simulink model "EVdemo_6"  (R2013b)
settings: Solver=FixedStepDiscrete  SolverMode=SingleTasking  StartTime=0.0  StopTime=650  FixedStep=4e-5  MaxStep=1e-5  RelTol=1e-3
InitFcn:
  | %EV_Param_Update
  | % update the number of strings (discretized)
  | numStrings = round(Opti_numStrings);
  | %disp(['Number of strings: ' num2str(numStrings)])
  | % update the effective capacity based on the number of strings
  | EV_Param.Battery_Det.Rated_Capacity = 28.5*numStrings; %A*hr
  | EV_Param.Battery_Det.DP = 1.5*fliplr([1500 1500 1600 1450 1325 1125 925 675 425 175 ])./8*EV_Param.Battery_Det.Rated_Capacity; % 8 comes from the 8Ahr rated batter data used (normalize and rescale to the rated capacity
  | EV_Param.Battery_Det.CP = fliplr([25 100 200 250 375 550 750 950 1125 1150])./8*EV_Param.Battery_Det.Rated_Capacity;
  | 
  | % update the number of cells in a string (discretized)
  | numSeriesCells = round(Opti_numSeriesCells);
  | %disp(['Number of cells in a string: ' num2str(numSeriesCells)])
  | % update the nominal string volage and charge deficit
  | EV_Param.Battery_Det.Nominal_Voltage = numSeriesCells*cellVolts;
  | BatteryParams(1).Qe_init = 0;%EV_Param.Battery_Det.Rated_Capacity*(1-EV_Param.Battery_Det.Initial_SOC/100); %Ampere*hours
  | 
  | % update the total number of cells, battery pack mass and total vehicle
  | % mass
  | total_cells = numSeriesCells*numStrings;
  | %disp(['Total Number of cells: ' num2str(total_cells)])
  | EV_Param.BatteryMass = BatteryParams(1).cell_mass*total_cells;
  | %disp(['Total Battery Pack Mass: ' num2str(EV_Param.BatteryMass)])
  | EV_Param.Vehicle.Mass = 1300+EV_Param.BatteryMass;
  | 
  | % update the driveline gear ratio
  | EV_Param.Vehicle.Engine_Vehicle_Gear_Ratio = Opti_Vehicle_Gear_Ratio;
  | %disp(['Driveline gear ratio: ' num2str(Opti_Vehicle_Gear_Ratio)])
StartFcn:
  | %tic;
StopFcn:
  | %toc;
  | %disp([Final SOC: ' num2str(SOC_final)])
  | %disp([Final Vehicle Error: ' num2str(normed_SQE_final)])
model workspace (MAT data in the model file):
  MCOS : class17 (value not decoded)
  MCOS : class17 (value not decoded)
values from neighbouring files (symbols this model uses):
  Drive_Cycle_Num = 8    [startDemo.m]
undefined symbols (not defined in the file or in its folder): Acc_Cmd, BatteryParams, Brake_Set, cell_area, ctrlConst, current_phase_a, Dec_Cmd, direct_current, DiscIntNeverNeededParam, electromagnetic_torque, HEV_Param, Ion, Kt_Temps, Lithium, Mech_Power_kW, Opti_numSeriesCells, Opti_numStrings, Opti_Vehicle_Gear_Ratio, paramVelocityI, paramVelocityP, paramVelocityPICurrentSat, pmsm, quadrature_current, RLoadLoss, rotor_velocity, sigbuilder_block, Ts, Veh_Spd_Ref
libraries: fl_lib x306, nesl_utility x100, LeadAcidBattery_lib x60, simulink x23, powerlib x16, sdl_lib x7, elec_lib x4, electricdrivelib x2, checkpacklib x2, CustomDriveline_lib x2, LiBatteryBlocks x1, Capacitors_lib x1
(part 6 of 7)

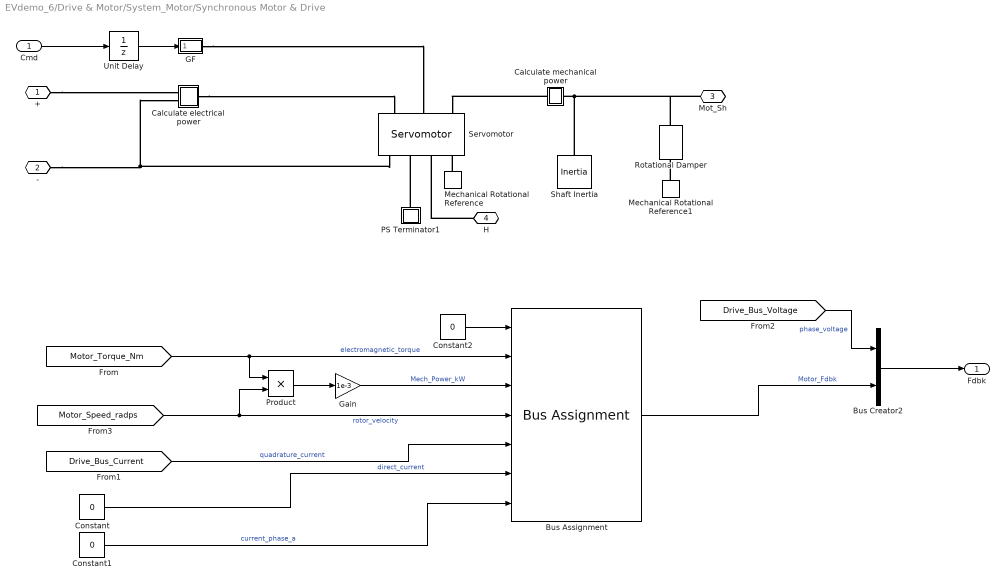
== system EVdemo_6/Drive & Motor/System_Motor/Synchronous Motor & Drive ==
  Cmd : Inport
  Bus Assignment : BusAssignment  AssignedSignals=electromagnetic_torque,Mech_Power_kW,rotor_velocity,quadrature_current,direct_current,current_phase_a
  Bus Creator2 : BusCreator  Inputs=2
  Calculate electrical power : Subsystem
      mask Display: disp('S')
  Calculate mechanical power : Subsystem
      mask Display: disp('S')
  Constant : Constant  Value=0  SampleTime=-1
  Constant1 : Constant  Value=0  SampleTime=-1
  Constant2 : Constant  Value=0  OutDataTypeStr=Bus: Motor_Fdbk  SampleTime=-1
  GF : Subsystem
      mask Display: disp('GF')
  Gain : Gain  Gain=1e-3
  Mechanical Rotational Reference : fl_lib/Mechanical/Rotational Elements/Mechanical Rotational Reference  t_Log=off  LocalVarNames=|t  LocalVarDescs=|t  LocalVarLogging=[]
  Mechanical Rotational Reference1 : fl_lib/Mechanical/Rotational Elements/Mechanical Rotational Reference  t_Log=off  LocalVarNames=|t  LocalVarDescs=|t  LocalVarLogging=0
  PS Terminator1 : Subsystem
      mask Display:
      | plot([0 0.9],[0.5 0.5]);
      | plot([0.5 0.9],[0.3 0.3]);
      | plot([0.5 0.9],[0.7 0.7]);
      | plot([0.9 0.9],[0.7 0.3]);
  Product : Product
  Rotational Damper : fl_lib/Mechanical/Rotational Elements/Rotational Damper  D=EV_Param.Motor.Damping N*m/(rad/s)  t_Log=off  w_Log=off  LocalVarNames=|t|w  LocalVarDescs=|t|w  LocalVarLogging=[0 0]
  Servomotor : elec_lib/Actuators & Drivers/Rotational Actuators/Servomotor  torque_speed_param=1  w_t=EV_Param.Motor.TorqSpdLUT.SpeedRPM rpm  T_t=EV_Param.Motor.TorqSpdLUT.TorqueNm N*m  torque_max=0.1 N*m  power_max=30 W  Tc=EV_Param.Motor.TorqueControl_TimeConst s  eff=EV_Param.Motor.Efficiency  w_eff=4000 rpm  T_eff=280 N*m  Piron=0 W  Pbase=0 W  Res=EV_Param.Motor.Series_Resistance Ohm  J=0 kg*m^2  lam=0 N*m/(rad/s)  speed0=0 rpm  LocalVarLogging=[]  alpha=0.00393 1/K  Tmeas=21 C  thermal_mass=10000 J/K  initial_temperature=21 C
  Shaft Inertia : fl_lib/Mechanical/Rotational Elements/Inertia  inertia=EV_Param.Motor.Shaft_Inertia kg*m^2  initial_velocity=0 rad/s  t_Log=off  LocalVarNames=|t  LocalVarDescs=|t  LocalVarLogging=0
  Unit Delay : UnitDelay  SampleTime=-1
  + : PMIOPort  Port=1  Side=Left
  - : PMIOPort  Port=2  Side=Left
  Mot_Sh : PMIOPort  Port=3  Side=Right
  H : PMIOPort  Port=4  Side=Left
  Fdbk : Outport
  wires:
  Unit Delay/1 -> GF/1(In1)
  Constant1/1 -> Bus Assignment/7  "current_phase_a"
  Constant/1 -> Bus Assignment/6  "direct_current"
  [Drive_Bus_Current] -> Bus Assignment/5  "quadrature_current"
  [Motor_Speed_radps] -> Bus Assignment/4, Product/2  "rotor_velocity"
  [Motor_Torque_Nm] -> Bus Assignment/2, Product/1  "electromagnetic_torque"
  Bus Creator2/1 -> Fdbk/1
  [Drive_Bus_Voltage] -> Bus Creator2/1  "phase_voltage"
  Cmd/1 -> Unit Delay/1
  Product/1 -> Gain/1
  Gain/1 -> Bus Assignment/3  "Mech_Power_kW"
  Constant2/1 -> Bus Assignment/1
  Bus Assignment/1 -> Bus Creator2/2  "Motor_Fdbk"
  connections:
  Mechanical Rotational Reference1/LConn1 -- Rotational Damper/RConn1
  +/RConn1 -- Calculate electrical power/LConn1
  Calculate electrical power/RConn1 -- Servomotor/LConn1
  Shaft Inertia/LConn1 -- Calculate mechanical power/RConn1 -- Rotational Damper/LConn1 -- Mot_Sh/RConn1
  PS Terminator1/LConn1 -- Servomotor/RConn2
  -/RConn1 -- Calculate electrical power/LConn2 -- Servomotor/RConn1
  GF/RConn1 -- Servomotor/LConn2
  Calculate mechanical power/LConn1 -- Servomotor/LConn3
  H/RConn1 -- Servomotor/RConn3
  Mechanical Rotational Reference/LConn1 -- Servomotor/RConn4

== system EVdemo_6/Drive & Motor/System_Motor/ZZZ_Background_Box ==

== system EVdemo_6/Operator Model/Accel_Cmd_Gen/Clamp ==
  preSat : Inport
  saturated : Inport  Port=2
  preIntegrator : Inport  Port=3
  AND : Logic  OutDataTypeStr=boolean
  Compare To Zero : simulink/Logic and Bit Operations/Compare To Zero  relop=<=  OutDataTypeStr=boolean
  Compare To Zero1 : simulink/Logic and Bit Operations/Compare To Zero  relop=<=  OutDataTypeStr=boolean
  Logical Operator : Logic  Operator=NXOR  AllPortsSameDT=off  OutDataTypeStr=boolean
  Clamp : Outport
  wires:
  AND/1 -> Clamp/1
  saturated/1 -> AND/2
  preIntegrator/1 -> Compare To Zero/1
  preSat/1 -> Compare To Zero1/1
  Logical Operator/1 -> AND/1
  Compare To Zero/1 -> Logical Operator/1
  Compare To Zero1/1 -> Logical Operator/2

== system EVdemo_6/Operator Model/Accel_Cmd_Gen/Convert_Data_Type ==
  In1 : Inport
  Data Type Conversion : DataTypeConversion  Priority=27
  Data Type Propagation : simulink/Signal Attributes/Data Type Propagation  Priority=24  PropDataType=fixdt(1, 16)  IfRefDouble=double  IfRefSingle=single  IsSigned=IsSigned1  NumBitsBase=NumBits1  NumBitsMult=1  NumBitsAdd=0  NumBitsAllowFinal=1:128  PropScaling=2^-10  ValuesUsedBestPrec=[5 -7]  SlopeBase=Slope1  SlopeMult=2  SlopeAdd=0  BiasBase=Bias1  BiasMult=1  BiasAdd=0
      settings: AttributesFormatString=-------------------------------\nDT = %<PropDataType>
  Out1 : Outport
  wires:
  In1/1 -> Data Type Propagation/2, Data Type Propagation/1, Data Type Conversion/1
  Data Type Conversion/1 -> Out1/1, Data Type Propagation/3

== system EVdemo_6/Operator Model/Accel_Cmd_Gen/Maintain_Range ==
  In1 : Inport
  Data Type Conversion : DataTypeConversion
  Data Type Propagation : simulink/Signal Attributes/Data Type Propagation  PropDataTypeMode=Specify via dialog  PropDataType=DT_PRECISION_LO  IfRefDouble=double  IfRefSingle=single  IsSigned=IsSigned1  NumBitsBase=NumBits1  NumBitsMult=0  NumBitsAdd=0  NumBitsAllowFinal=1:128  PropScaling=2^-10  ValuesUsedBestPrec=[5 -7]  SlopeBase=PosRange1  SlopeMult=1  SlopeAdd=0  BiasBase=Bias1  BiasMult=1  BiasAdd=0
      settings: AttributesFormatString=-------------------------------\nDT = %<PropDataType>
  Out1 : Outport
  wires:
  In1/1 -> Data Type Propagation/2, Data Type Propagation/1, Data Type Conversion/1
  Data Type Conversion/1 -> Out1/1, Data Type Propagation/3

== system EVdemo_6/Operator Model/Accel_Cmd_Gen/PI_Sat ==
  In1 : Inport
  Constant : Constant  Value=0
  Dynamic Saturation : Subsystem
      mask Display: plot([0.15 0.85],[.5 .5],[.5 .5],[0.05 0.95],0.15+0.7*[0 .25 .75 1],0.05+0.9*[.25 .25 .75 .75]);
  PI_Sat : Constant  Value=EV_Param.Control.Veh_Spd.Sat  PreserveConstantTs=on
  Out1 : Outport
  saturated : Outport  Port=2
  wires:
  Dynamic Saturation/2(sat_mode) -> saturated/1
  Dynamic Saturation/1(y) -> Out1/1
  PI_Sat/1 -> Dynamic Saturation/1(up)
  In1/1 -> Dynamic Saturation/2(u)
  Constant/1 -> Dynamic Saturation/3(lo)

== system EVdemo_6/Operator Model/Brake_Cmd_Gen/Clamp ==
  preSat : Inport
  saturated : Inport  Port=2
  preIntegrator : Inport  Port=3
  AND : Logic  OutDataTypeStr=boolean
  Compare To Zero : simulink/Logic and Bit Operations/Compare To Zero  relop=<=  OutDataTypeStr=boolean
  Compare To Zero1 : simulink/Logic and Bit Operations/Compare To Zero  relop=<=  OutDataTypeStr=boolean
  Logical Operator : Logic  Operator=NXOR  AllPortsSameDT=off  OutDataTypeStr=boolean
  Clamp : Outport
  wires:
  Compare To Zero1/1 -> Logical Operator/2
  Compare To Zero/1 -> Logical Operator/1
  Logical Operator/1 -> AND/1
  preSat/1 -> Compare To Zero1/1
  preIntegrator/1 -> Compare To Zero/1
  saturated/1 -> AND/2
  AND/1 -> Clamp/1

== system EVdemo_6/Operator Model/Brake_Cmd_Gen/Convert_Data_Type ==
  In1 : Inport
  Data Type Conversion : DataTypeConversion  Priority=27
  Data Type Propagation : simulink/Signal Attributes/Data Type Propagation  Priority=24  PropDataType=fixdt(1, 16)  IfRefDouble=double  IfRefSingle=single  IsSigned=IsSigned1  NumBitsBase=NumBits1  NumBitsMult=1  NumBitsAdd=0  NumBitsAllowFinal=1:128  PropScaling=2^-10  ValuesUsedBestPrec=[5 -7]  SlopeBase=Slope1  SlopeMult=2  SlopeAdd=0  BiasBase=Bias1  BiasMult=1  BiasAdd=0
      settings: AttributesFormatString=-------------------------------\nDT = %<PropDataType>
  Out1 : Outport
  wires:
  Data Type Conversion/1 -> Data Type Propagation/3, Out1/1
  In1/1 -> Data Type Conversion/1, Data Type Propagation/1, Data Type Propagation/2

== system EVdemo_6/Operator Model/Brake_Cmd_Gen/Maintain_Range ==
  In1 : Inport
  Data Type Conversion : DataTypeConversion
  Data Type Propagation : simulink/Signal Attributes/Data Type Propagation  PropDataTypeMode=Specify via dialog  PropDataType=DT_PRECISION_LO  IfRefDouble=double  IfRefSingle=single  IsSigned=IsSigned1  NumBitsBase=NumBits1  NumBitsMult=0  NumBitsAdd=0  NumBitsAllowFinal=1:128  PropScaling=2^-10  ValuesUsedBestPrec=[5 -7]  SlopeBase=PosRange1  SlopeMult=1  SlopeAdd=0  BiasBase=Bias1  BiasMult=1  BiasAdd=0
      settings: AttributesFormatString=-------------------------------\nDT = %<PropDataType>
  Out1 : Outport
  wires:
  Data Type Conversion/1 -> Data Type Propagation/3, Out1/1
  In1/1 -> Data Type Conversion/1, Data Type Propagation/1, Data Type Propagation/2

== system EVdemo_6/Operator Model/Brake_Cmd_Gen/PI_Sat ==
  In1 : Inport
  Constant : Constant  Value=0
  Dynamic Saturation : Subsystem
      mask Display: plot([0.15 0.85],[.5 .5],[.5 .5],[0.05 0.95],0.15+0.7*[0 .25 .75 1],0.05+0.9*[.25 .25 .75 .75]);
  PI_Sat : Constant  Value=-EV_Param.Control.Veh_Brake.Sat  PreserveConstantTs=on
  Out1 : Outport
  saturated : Outport  Port=2
  wires:
  Constant/1 -> Dynamic Saturation/1(up)
  In1/1 -> Dynamic Saturation/2(u)
  PI_Sat/1 -> Dynamic Saturation/3(lo)
  Dynamic Saturation/1(y) -> Out1/1
  Dynamic Saturation/2(sat_mode) -> saturated/1

== system EVdemo_6/Vehicle/Full/2nd Order LP Filter (Butterworth) ==
  u : Inport
  Spd_Err_Filt_BW [rad/s] : Inport  Port=2
  -1 : Gain  Gain=-1
  -1.4142/(Spd_Err_Filt_BW) : Gain  Gain=-1.4142
  Add4 : Sum  Inputs=+++
  Compare To Zero : simulink/Logic and Bit Operations/Compare To Zero  relop=<=  OutDataTypeStr=uint8
  Discrete-Time Integrator : DiscreteIntegrator  ExternalReset=rising  SampleTime=DT  ICPrevOutput=DiscIntNeverNeededParam  ICPrevScaledInput=DiscIntNeverNeededParam
  Discrete-Time Integrator1 : DiscreteIntegrator  ExternalReset=rising  SampleTime=DT  ICPrevOutput=DiscIntNeverNeededParam  ICPrevScaledInput=DiscIntNeverNeededParam
  Math Function : Math  Operator=square  SaturateOnIntegerOverflow=on
  Product : Product  RndMeth=Zero
  Product1 : Product  Inputs=*/  RndMeth=Zero
  Saturation1 : Saturate  UpperLimit=2*pi*5000  LowerLimit=.001
  y : Outport
  wires:
  Add4/1 -> Product/2
  Discrete-Time Integrator/1 -> Product1/1, Discrete-Time Integrator1/1  "X_1"
  Discrete-Time Integrator1/1 -> -1/1, y/1  "x_2"
  -1.4142/(Spd_Err_Filt_BW)/1 -> Add4/3
  -1/1 -> Add4/2
  Product/1 -> Discrete-Time Integrator/1  "x_0"
  u/1 -> Add4/1
  Math Function/1 -> Product/1, Compare To Zero/1
  Spd_Err_Filt_BW [rad/s]/1 -> Saturation1/1
  Product1/1 -> -1.4142/(Spd_Err_Filt_BW)/1
  Compare To Zero/1 -> Discrete-Time Integrator/2, Discrete-Time Integrator1/2
  Saturation1/1 -> Math Function/1, Product1/2

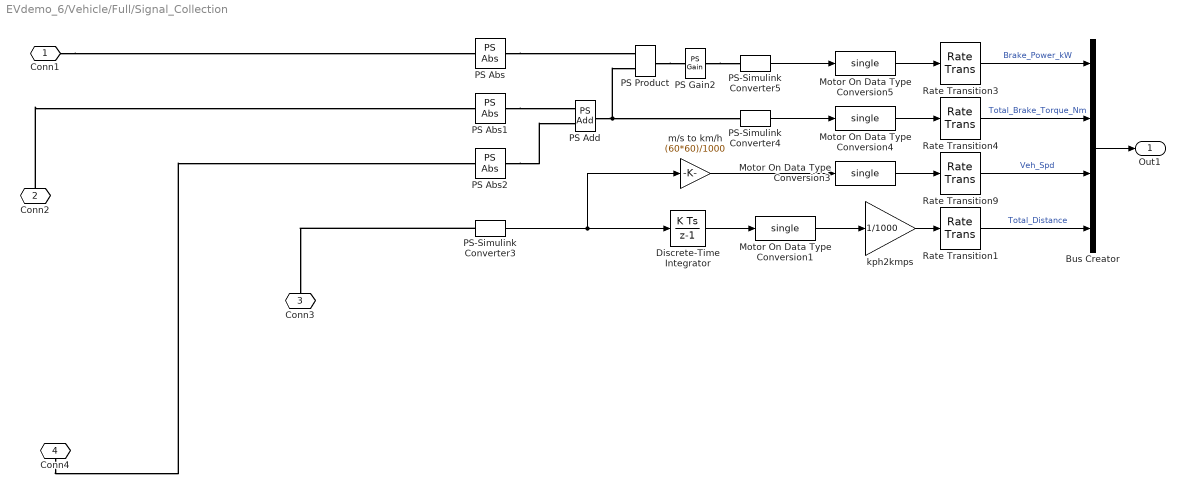
== system EVdemo_6/Vehicle/Full/Signal_Collection ==
  Bus Creator : BusCreator
  Discrete-Time Integrator : DiscreteIntegrator  SampleTime=-1  ICPrevOutput=DiscIntNeverNeededParam  ICPrevScaledInput=DiscIntNeverNeededParam
  Motor On Data Type Conversion{1,3..5} (4 alike) : DataTypeConversion  OutDataTypeStr=single
  PS Abs : fl_lib/Physical Signals/Nonlinear Operators/PS Abs  LocalVarLogging=[]
  PS Abs1 : fl_lib/Physical Signals/Nonlinear Operators/PS Abs  LocalVarLogging=[]
  PS Abs2 : fl_lib/Physical Signals/Nonlinear Operators/PS Abs  LocalVarLogging=[]
  PS Add : fl_lib/Physical Signals/Functions/PS Add  LocalVarLogging=[]
  PS Gain2 : fl_lib/Physical Signals/Functions/PS Gain  gain=1e-3  LocalVarLogging=[]
  PS Product : fl_lib/Physical Signals/Functions/PS Product  LocalVarLogging=[]
  PS-Simulink Converter3 : nesl_utility/PS-Simulink Converter  PhysicalDomain=network_engine_domain  SubClassName=ps_output  LeftPortType=input  RightPortType=output  PseudoPeriodic=off  Frequencies=[]  Unit=m/s  AffineConversion=off
  PS-Simulink Converter4 : nesl_utility/PS-Simulink Converter  PhysicalDomain=network_engine_domain  SubClassName=ps_output  LeftPortType=input  RightPortType=output  PseudoPeriodic=off  Frequencies=[]  Unit=m/s  AffineConversion=off
  PS-Simulink Converter5 : nesl_utility/PS-Simulink Converter  PhysicalDomain=network_engine_domain  SubClassName=ps_output  LeftPortType=input  RightPortType=output  PseudoPeriodic=off  Frequencies=[]  Unit=m/s  AffineConversion=off
  Rate Transition{1,3..4,9} (4 alike) : RateTransition  OutPortSampleTime=.01
  kph2kmps : Gain  Gain=1/1000
  m/s to km/h : Gain  Gain=(60*60)/1000
  Conn1 : PMIOPort  Port=1  Side=Left
  Conn2 : PMIOPort  Port=2  Side=Left
  Conn3 : PMIOPort  Port=3  Side=Left
  Conn4 : PMIOPort  Port=4  Side=Left
  Out1 : Outport
  wires:
  PS-Simulink Converter4/1 -> Motor On Data Type Conversion4/1
  PS-Simulink Converter5/1 -> Motor On Data Type Conversion5/1
  Rate Transition3/1 -> Bus Creator/1  "Brake_Power_kW"
  Rate Transition4/1 -> Bus Creator/2  "Total_Brake_Torque_Nm"
  Motor On Data Type Conversion4/1 -> Rate Transition4/1
  Motor On Data Type Conversion5/1 -> Rate Transition3/1
  Discrete-Time Integrator/1 -> Motor On Data Type Conversion1/1
  m/s to km/h/1 -> Motor On Data Type Conversion3/1
  Motor On Data Type Conversion3/1 -> Rate Transition9/1
  kph2kmps/1 -> Rate Transition1/1
  Rate Transition1/1 -> Bus Creator/4  "Total_Distance"
  Bus Creator/1 -> Out1/1
  Motor On Data Type Conversion1/1 -> kph2kmps/1
  Rate Transition9/1 -> Bus Creator/3  "Veh_Spd"
  PS-Simulink Converter3/1 -> m/s to km/h/1, Discrete-Time Integrator/1
  connections:
  PS Abs/RConn1 -- PS Product/LConn1
  PS Product/RConn1 -- PS Gain2/LConn1
  PS Gain2/RConn1 -- PS-Simulink Converter5/LConn1
  PS Abs1/RConn1 -- PS Add/LConn1
  PS Abs2/RConn1 -- PS Add/LConn2
  Conn1/RConn1 -- PS Abs/LConn1
  PS Add/RConn1 -- PS Product/LConn2 -- PS-Simulink Converter4/LConn1
  Conn2/RConn1 -- PS Abs1/LConn1
  Conn4/RConn1 -- PS Abs2/LConn1
  PS-Simulink Converter3/LConn1 -- Conn3/RConn1

== system EVdemo_6/Vehicle/Full/Vehicle Speed, Power ==
  Ideal Rotational Motion Sensor : fl_lib/Mechanical/Mechanical Sensors/Ideal Rotational Motion Sensor  offset=0 rad  w_Log=off  t_Log=off  phi_Log=off  LocalVarNames=|w|t|phi  LocalVarDescs=|w|t|phi  LocalVarLogging=[0 0 0]
  Ideal Torque Sensor : fl_lib/Mechanical/Mechanical Sensors/Ideal Torque Sensor  w_Log=off  t_Log=off  LocalVarNames=|w|t  LocalVarDescs=|w|t  LocalVarLogging=[0 0]
  Mechanical Rotational Reference : fl_lib/Mechanical/Rotational Elements/Mechanical Rotational Reference  t_Log=off  LocalVarNames=|t  LocalVarDescs=|t  LocalVarLogging=0
  PS-Simulink Converter : nesl_utility/PS-Simulink Converter  PhysicalDomain=network_engine_domain  SubClassName=ps_output  LeftPortType=input  RightPortType=output  PseudoPeriodic=off  Frequencies=[]  Unit=N*m  AffineConversion=off
  PS-Simulink Converter1 : nesl_utility/PS-Simulink Converter  PhysicalDomain=network_engine_domain  SubClassName=ps_output  LeftPortType=input  RightPortType=output  PseudoPeriodic=off  Frequencies=[]  Unit=rad/s  AffineConversion=off
  Product : Product  RndMeth=Zero
  W2kW : Gain  Gain=0.001
  B : PMIOPort  Port=1  Side=Left
  F : PMIOPort  Port=2  Side=Right
  tag scope: Pm_vehicle=global
  wires:
  PS-Simulink Converter1/1 -> Product/2
  PS-Simulink Converter/1 -> Product/1
  Product/1 -> W2kW/1
  W2kW/1 -> [Pm_vehicle]
  connections:
  PS-Simulink Converter1/LConn1 -- Ideal Rotational Motion Sensor/RConn2
  PS-Simulink Converter/LConn1 -- Ideal Torque Sensor/RConn2
  B/RConn1 -- Ideal Torque Sensor/LConn1
  Ideal Torque Sensor/RConn1 -- F/RConn1 -- Ideal Rotational Motion Sensor/LConn1
  Mechanical Rotational Reference/LConn1 -- Ideal Rotational Motion Sensor/RConn1

== system EVdemo_6/Vehicle/Simple/Aerodynamic Drag ==
  Cd1 : fl_lib/Physical Signals/Functions/PS Gain  gain=Cd  LocalVarLogging=[]
  PS Math Function : fl_lib/Physical Signals/Functions/PS Math Function  fcn_choice=7  LocalVarLogging=[]
  PS Product : fl_lib/Physical Signals/Functions/PS Product  LocalVarLogging=[]
  PS Sign : fl_lib/Physical Signals/Nonlinear Operators/PS Sign  LocalVarLogging=[]
  half1 : fl_lib/Physical Signals/Functions/PS Gain  gain=1/2  LocalVarLogging=[]
  kph to mps1 : fl_lib/Physical Signals/Functions/PS Gain  gain=1/3.6  LocalVarLogging=[]
  radius1 : fl_lib/Physical Signals/Functions/PS Gain  gain=-radius  LocalVarLogging=[]
  Conn1 : PMIOPort  Port=1  Side=Left
  Conn2 : PMIOPort  Port=2  Side=Right
  connections:
  PS Sign/RConn1 -- PS Product/LConn2
  radius1/LConn1 -- Cd1/RConn1
  radius1/RConn1 -- PS Product/LConn1
  Cd1/LConn1 -- half1/RConn1
  PS Math Function/LConn1 -- kph to mps1/RConn1
  half1/LConn1 -- PS Math Function/RConn1
  kph to mps1/LConn1 -- PS Sign/LConn1 -- Conn1/RConn1
  Conn2/RConn1 -- PS Product/RConn1

== system EVdemo_6/Vehicle/Simple/Vehicle Speed, Power ==
  Ideal Rotational Motion Sensor : fl_lib/Mechanical/Mechanical Sensors/Ideal Rotational Motion Sensor  offset=0 rad  w_Log=off  t_Log=off  phi_Log=off  LocalVarNames=|w|t|phi  LocalVarDescs=|w|t|phi  LocalVarLogging=[0 0 0]
  Ideal Torque Sensor : fl_lib/Mechanical/Mechanical Sensors/Ideal Torque Sensor  w_Log=off  t_Log=off  LocalVarNames=|w|t  LocalVarDescs=|w|t  LocalVarLogging=[0 0]
  Mechanical Rotational Reference : fl_lib/Mechanical/Rotational Elements/Mechanical Rotational Reference  t_Log=off  LocalVarNames=|t  LocalVarDescs=|t  LocalVarLogging=0
  PS-Simulink Converter : nesl_utility/PS-Simulink Converter  PhysicalDomain=network_engine_domain  SubClassName=ps_output  LeftPortType=input  RightPortType=output  PseudoPeriodic=off  Frequencies=[]  Unit=N*m  AffineConversion=off
  PS-Simulink Converter1 : nesl_utility/PS-Simulink Converter  PhysicalDomain=network_engine_domain  SubClassName=ps_output  LeftPortType=input  RightPortType=output  PseudoPeriodic=off  Frequencies=[]  Unit=rad/s  AffineConversion=off
  Product : Product  RndMeth=Zero
  W2kW : Gain  Gain=0.001
  rad/s to km/h : fl_lib/Physical Signals/Functions/PS Gain  gain=radius*3.6  LocalVarLogging=[]
  B : PMIOPort  Port=1  Side=Left
  F : PMIOPort  Port=2  Side=Left
  Speed : PMIOPort  Port=3  Side=Right
  tag scope: Pm_vehicle=global
  wires:
  W2kW/1 -> [Pm_vehicle]
  Product/1 -> W2kW/1
  PS-Simulink Converter/1 -> Product/1
  PS-Simulink Converter1/1 -> Product/2
  connections:
  Mechanical Rotational Reference/LConn1 -- Ideal Rotational Motion Sensor/RConn1
  Ideal Rotational Motion Sensor/LConn1 -- F/RConn1 -- Ideal Torque Sensor/RConn1
  B/RConn1 -- Ideal Torque Sensor/LConn1
  PS-Simulink Converter/LConn1 -- Ideal Torque Sensor/RConn2
  rad/s to km/h/LConn1 -- Ideal Rotational Motion Sensor/RConn2 -- PS-Simulink Converter1/LConn1
  Speed/RConn1 -- rad/s to km/h/RConn1

== system EVdemo_6/Battery/Cells/Battery cell1/ DOC  ==
  PS-Simulink Converter1 : nesl_utility/PS-Simulink Converter  PhysicalDomain=network_engine_domain  SubClassName=ps_output  LeftPortType=input  RightPortType=output  PseudoPeriodic=off  Frequencies=[]  Unit=1  AffineConversion=off
  PS : PMIOPort  Port=1  Side=Left
  tag scope: DOC=global
  wires:
  PS-Simulink Converter1/1 -> [DOC]
  connections:
  PS/RConn1 -- PS-Simulink Converter1/LConn1

== system EVdemo_6/Battery/Cells/Battery cell1/ SOC  ==
  PS-Simulink Converter1 : nesl_utility/PS-Simulink Converter  PhysicalDomain=network_engine_domain  SubClassName=ps_output  LeftPortType=input  RightPortType=output  PseudoPeriodic=off  Frequencies=[]  Unit=1  AffineConversion=off
  PS : PMIOPort  Port=1  Side=Left
  tag scope: SOC=global
  wires:
  PS-Simulink Converter1/1 -> [SOC]
  connections:
  PS/RConn1 -- PS-Simulink Converter1/LConn1

== system EVdemo_6/Battery/Cells/Battery cell1/T ==
  PS-Simulink Converter1 : nesl_utility/PS-Simulink Converter  PhysicalDomain=network_engine_domain  SubClassName=ps_output  LeftPortType=input  RightPortType=output  PseudoPeriodic=off  Frequencies=[]  Unit=C  AffineConversion=on
  PS : PMIOPort  Port=1  Side=Left
  tag scope: Batt_Cell_Temp=global
  wires:
  PS-Simulink Converter1/1 -> [Batt_Cell_Temp]
  connections:
  PS/RConn1 -- PS-Simulink Converter1/LConn1

== system EVdemo_6/Battery/Cells/Battery cell1/Thermal Model ==
  Battery thermal mass : fl_lib/Thermal/Thermal Elements/Thermal Mass  mass=1 kg  sp_heat=HEV_Param.Battery_Cell.Ctheta J/kg/K  init_temp=HEV_Param.Battery_Cell.theta_init+273 K  Q_Log=off  LocalVarNames=|heat_flow|temperature  LocalVarDescs=|Heat flow (J/s)|Mass temperature (K)  LocalVarLogging=[0 0]
  Ideal Temperature Sensor : fl_lib/Thermal/Thermal Sensors/Ideal Temperature Sensor  Qs_Log=off  Ts_Log=off  LocalVarNames=|Qs|Ts  LocalVarDescs=|Qs|Ts  LocalVarLogging=[]
  Ideal Heat Flow Source : fl_lib/Thermal/Thermal Sources/Ideal Heat Flow Source  Q_Log=off  T_Log=off  LocalVarNames=|heat_flow|T_differential  LocalVarDescs=|Heat flow through the source (J/s)|Temperature differential across the source (K)  LocalVarLogging=[0 0]
  Kt as a function of temperature : fl_lib/Physical Signals/Lookup Tables/PS Lookup Table (1D)  x_t=[HEV_Param.Battery_Cell.theta_f,HEV_Param.Battery_Cell. Kt_Temps]+273  y_t=[0 HEV_Param.Battery_Cell.Kt]  interp_method=1  extrap_method=1  LocalVarLogging=[]
  Thermal Reference1 : fl_lib/Thermal/Thermal Elements/Thermal Reference  Q_Log=off  LocalVarNames=|Q  LocalVarDescs=|Q  LocalVarLogging=[]
  Thermal Reference2 : fl_lib/Thermal/Thermal Elements/Thermal Reference  Q_Log=off  LocalVarNames=|Q  LocalVarDescs=|Q  LocalVarLogging=[]
  Ps : PMIOPort  Tag=PMCPort  Port=1  Side=Left
  H : PMIOPort  Tag=PMCPort  Port=2  Side=Left
  Kt : PMIOPort  Tag=PMCPort  Port=3  Side=Right
  T : PMIOPort  Tag=PMCPort  Port=4  Side=Right
  connections:
  Ideal Heat Flow Source/RConn1 -- Ps/RConn1
  Kt/RConn1 -- Kt as a function of temperature/RConn1
  Battery thermal mass/LConn1 -- Ideal Heat Flow Source/LConn1 -- Ideal Temperature Sensor/LConn1 -- H/RConn1
  Thermal Reference1/LConn1 -- Ideal Heat Flow Source/RConn2
  T/RConn1 -- Kt as a function of temperature/LConn1 -- Ideal Temperature Sensor/RConn2
  Ideal Temperature Sensor/RConn1 -- Thermal Reference2/LConn1

== system EVdemo_6/Battery/Cells/Battery cell10/Thermal Model ==
  Battery thermal mass : fl_lib/Thermal/Thermal Elements/Thermal Mass  mass=1 kg  sp_heat=HEV_Param.Battery_Cell.Ctheta J/kg/K  init_temp=HEV_Param.Battery_Cell.theta_init+273 K  Q_Log=off  LocalVarNames=|heat_flow|temperature  LocalVarDescs=|Heat flow (J/s)|Mass temperature (K)  LocalVarLogging=[0 0]
  Ideal Temperature Sensor : fl_lib/Thermal/Thermal Sensors/Ideal Temperature Sensor  Qs_Log=off  Ts_Log=off  LocalVarNames=|Qs|Ts  LocalVarDescs=|Qs|Ts  LocalVarLogging=[]
  Ideal Heat Flow Source : fl_lib/Thermal/Thermal Sources/Ideal Heat Flow Source  Q_Log=off  T_Log=off  LocalVarNames=|heat_flow|T_differential  LocalVarDescs=|Heat flow through the source (J/s)|Temperature differential across the source (K)  LocalVarLogging=[0 0]
  Kt as a function of temperature : fl_lib/Physical Signals/Lookup Tables/PS Lookup Table (1D)  x_t=[HEV_Param.Battery_Cell.theta_f,HEV_Param.Battery_Cell. Kt_Temps]+273  y_t=[0 HEV_Param.Battery_Cell.Kt]  interp_method=1  extrap_method=1  LocalVarLogging=[]
  Thermal Reference1 : fl_lib/Thermal/Thermal Elements/Thermal Reference  Q_Log=off  LocalVarNames=|Q  LocalVarDescs=|Q  LocalVarLogging=[]
  Thermal Reference2 : fl_lib/Thermal/Thermal Elements/Thermal Reference  Q_Log=off  LocalVarNames=|Q  LocalVarDescs=|Q  LocalVarLogging=[]
  Ps : PMIOPort  Tag=PMCPort  Port=1  Side=Left
  H : PMIOPort  Tag=PMCPort  Port=2  Side=Left
  Kt : PMIOPort  Tag=PMCPort  Port=3  Side=Right
  T : PMIOPort  Tag=PMCPort  Port=4  Side=Right
  connections:
  Ideal Heat Flow Source/RConn1 -- Ps/RConn1
  Kt/RConn1 -- Kt as a function of temperature/RConn1
  Battery thermal mass/LConn1 -- Ideal Heat Flow Source/LConn1 -- Ideal Temperature Sensor/LConn1 -- H/RConn1
  Thermal Reference1/LConn1 -- Ideal Heat Flow Source/RConn2
  T/RConn1 -- Kt as a function of temperature/LConn1 -- Ideal Temperature Sensor/RConn2
  Ideal Temperature Sensor/RConn1 -- Thermal Reference2/LConn1

== system EVdemo_6/Battery/Cells/Battery cell2/Thermal Model ==
  Battery thermal mass : fl_lib/Thermal/Thermal Elements/Thermal Mass  mass=1 kg  sp_heat=HEV_Param.Battery_Cell.Ctheta J/kg/K  init_temp=HEV_Param.Battery_Cell.theta_init+273 K  Q_Log=off  LocalVarNames=|heat_flow|temperature  LocalVarDescs=|Heat flow (J/s)|Mass temperature (K)  LocalVarLogging=[0 0]
  Ideal Temperature Sensor : fl_lib/Thermal/Thermal Sensors/Ideal Temperature Sensor  Qs_Log=off  Ts_Log=off  LocalVarNames=|Qs|Ts  LocalVarDescs=|Qs|Ts  LocalVarLogging=[]
  Ideal Heat Flow Source : fl_lib/Thermal/Thermal Sources/Ideal Heat Flow Source  Q_Log=off  T_Log=off  LocalVarNames=|heat_flow|T_differential  LocalVarDescs=|Heat flow through the source (J/s)|Temperature differential across the source (K)  LocalVarLogging=[0 0]
  Kt as a function of temperature : fl_lib/Physical Signals/Lookup Tables/PS Lookup Table (1D)  x_t=[HEV_Param.Battery_Cell.theta_f,HEV_Param.Battery_Cell. Kt_Temps]+273  y_t=[0 HEV_Param.Battery_Cell.Kt]  interp_method=1  extrap_method=1  LocalVarLogging=[]
  Thermal Reference1 : fl_lib/Thermal/Thermal Elements/Thermal Reference  Q_Log=off  LocalVarNames=|Q  LocalVarDescs=|Q  LocalVarLogging=[]
  Thermal Reference2 : fl_lib/Thermal/Thermal Elements/Thermal Reference  Q_Log=off  LocalVarNames=|Q  LocalVarDescs=|Q  LocalVarLogging=[]
  Ps : PMIOPort  Tag=PMCPort  Port=1  Side=Left
  H : PMIOPort  Tag=PMCPort  Port=2  Side=Left
  Kt : PMIOPort  Tag=PMCPort  Port=3  Side=Right
  T : PMIOPort  Tag=PMCPort  Port=4  Side=Right
  connections:
  Ideal Temperature Sensor/RConn1 -- Thermal Reference2/LConn1
  Ideal Temperature Sensor/RConn2 -- Kt as a function of temperature/LConn1 -- T/RConn1
  Thermal Reference1/LConn1 -- Ideal Heat Flow Source/RConn2
  H/RConn1 -- Ideal Temperature Sensor/LConn1 -- Ideal Heat Flow Source/LConn1 -- Battery thermal mass/LConn1
  Kt/RConn1 -- Kt as a function of temperature/RConn1
  Ideal Heat Flow Source/RConn1 -- Ps/RConn1

== system EVdemo_6/Battery/Cells/Battery cell3/Thermal Model ==
  Battery thermal mass : fl_lib/Thermal/Thermal Elements/Thermal Mass  mass=1 kg  sp_heat=HEV_Param.Battery_Cell.Ctheta J/kg/K  init_temp=HEV_Param.Battery_Cell.theta_init+273 K  Q_Log=off  LocalVarNames=|heat_flow|temperature  LocalVarDescs=|Heat flow (J/s)|Mass temperature (K)  LocalVarLogging=[0 0]
  Ideal Temperature Sensor : fl_lib/Thermal/Thermal Sensors/Ideal Temperature Sensor  Qs_Log=off  Ts_Log=off  LocalVarNames=|Qs|Ts  LocalVarDescs=|Qs|Ts  LocalVarLogging=[]
  Ideal Heat Flow Source : fl_lib/Thermal/Thermal Sources/Ideal Heat Flow Source  Q_Log=off  T_Log=off  LocalVarNames=|heat_flow|T_differential  LocalVarDescs=|Heat flow through the source (J/s)|Temperature differential across the source (K)  LocalVarLogging=[0 0]
  Kt as a function of temperature : fl_lib/Physical Signals/Lookup Tables/PS Lookup Table (1D)  x_t=[HEV_Param.Battery_Cell.theta_f,HEV_Param.Battery_Cell. Kt_Temps]+273  y_t=[0 HEV_Param.Battery_Cell.Kt]  interp_method=1  extrap_method=1  LocalVarLogging=[]
  Thermal Reference1 : fl_lib/Thermal/Thermal Elements/Thermal Reference  Q_Log=off  LocalVarNames=|Q  LocalVarDescs=|Q  LocalVarLogging=[]
  Thermal Reference2 : fl_lib/Thermal/Thermal Elements/Thermal Reference  Q_Log=off  LocalVarNames=|Q  LocalVarDescs=|Q  LocalVarLogging=[]
  Ps : PMIOPort  Tag=PMCPort  Port=1  Side=Left
  H : PMIOPort  Tag=PMCPort  Port=2  Side=Left
  Kt : PMIOPort  Tag=PMCPort  Port=3  Side=Right
  T : PMIOPort  Tag=PMCPort  Port=4  Side=Right
  connections:
  Ideal Heat Flow Source/RConn1 -- Ps/RConn1
  Kt/RConn1 -- Kt as a function of temperature/RConn1
  Battery thermal mass/LConn1 -- Ideal Heat Flow Source/LConn1 -- Ideal Temperature Sensor/LConn1 -- H/RConn1
  Thermal Reference1/LConn1 -- Ideal Heat Flow Source/RConn2
  T/RConn1 -- Kt as a function of temperature/LConn1 -- Ideal Temperature Sensor/RConn2
  Ideal Temperature Sensor/RConn1 -- Thermal Reference2/LConn1

== system EVdemo_6/Battery/Cells/Battery cell4/Thermal Model ==
  Battery thermal mass : fl_lib/Thermal/Thermal Elements/Thermal Mass  mass=1 kg  sp_heat=HEV_Param.Battery_Cell.Ctheta J/kg/K  init_temp=HEV_Param.Battery_Cell.theta_init+273 K  Q_Log=off  LocalVarNames=|heat_flow|temperature  LocalVarDescs=|Heat flow (J/s)|Mass temperature (K)  LocalVarLogging=[0 0]
  Ideal Temperature Sensor : fl_lib/Thermal/Thermal Sensors/Ideal Temperature Sensor  Qs_Log=off  Ts_Log=off  LocalVarNames=|Qs|Ts  LocalVarDescs=|Qs|Ts  LocalVarLogging=[]
  Ideal Heat Flow Source : fl_lib/Thermal/Thermal Sources/Ideal Heat Flow Source  Q_Log=off  T_Log=off  LocalVarNames=|heat_flow|T_differential  LocalVarDescs=|Heat flow through the source (J/s)|Temperature differential across the source (K)  LocalVarLogging=[0 0]
  Kt as a function of temperature : fl_lib/Physical Signals/Lookup Tables/PS Lookup Table (1D)  x_t=[HEV_Param.Battery_Cell.theta_f,HEV_Param.Battery_Cell. Kt_Temps]+273  y_t=[0 HEV_Param.Battery_Cell.Kt]  interp_method=1  extrap_method=1  LocalVarLogging=[]
  Thermal Reference1 : fl_lib/Thermal/Thermal Elements/Thermal Reference  Q_Log=off  LocalVarNames=|Q  LocalVarDescs=|Q  LocalVarLogging=[]
  Thermal Reference2 : fl_lib/Thermal/Thermal Elements/Thermal Reference  Q_Log=off  LocalVarNames=|Q  LocalVarDescs=|Q  LocalVarLogging=[]
  Ps : PMIOPort  Tag=PMCPort  Port=1  Side=Left
  H : PMIOPort  Tag=PMCPort  Port=2  Side=Left
  Kt : PMIOPort  Tag=PMCPort  Port=3  Side=Right
  T : PMIOPort  Tag=PMCPort  Port=4  Side=Right
  connections:
  Ideal Heat Flow Source/RConn1 -- Ps/RConn1
  Kt/RConn1 -- Kt as a function of temperature/RConn1
  Battery thermal mass/LConn1 -- Ideal Heat Flow Source/LConn1 -- Ideal Temperature Sensor/LConn1 -- H/RConn1
  Thermal Reference1/LConn1 -- Ideal Heat Flow Source/RConn2
  T/RConn1 -- Kt as a function of temperature/LConn1 -- Ideal Temperature Sensor/RConn2
  Ideal Temperature Sensor/RConn1 -- Thermal Reference2/LConn1

== system EVdemo_6/Battery/Cells/Battery cell5/Thermal Model ==
  Battery thermal mass : fl_lib/Thermal/Thermal Elements/Thermal Mass  mass=1 kg  sp_heat=HEV_Param.Battery_Cell.Ctheta J/kg/K  init_temp=HEV_Param.Battery_Cell.theta_init+273 K  Q_Log=off  LocalVarNames=|heat_flow|temperature  LocalVarDescs=|Heat flow (J/s)|Mass temperature (K)  LocalVarLogging=[0 0]
  Ideal Temperature Sensor : fl_lib/Thermal/Thermal Sensors/Ideal Temperature Sensor  Qs_Log=off  Ts_Log=off  LocalVarNames=|Qs|Ts  LocalVarDescs=|Qs|Ts  LocalVarLogging=[]
  Ideal Heat Flow Source : fl_lib/Thermal/Thermal Sources/Ideal Heat Flow Source  Q_Log=off  T_Log=off  LocalVarNames=|heat_flow|T_differential  LocalVarDescs=|Heat flow through the source (J/s)|Temperature differential across the source (K)  LocalVarLogging=[0 0]
  Kt as a function of temperature : fl_lib/Physical Signals/Lookup Tables/PS Lookup Table (1D)  x_t=[HEV_Param.Battery_Cell.theta_f,HEV_Param.Battery_Cell. Kt_Temps]+273  y_t=[0 HEV_Param.Battery_Cell.Kt]  interp_method=1  extrap_method=1  LocalVarLogging=[]
  Thermal Reference1 : fl_lib/Thermal/Thermal Elements/Thermal Reference  Q_Log=off  LocalVarNames=|Q  LocalVarDescs=|Q  LocalVarLogging=[]
  Thermal Reference2 : fl_lib/Thermal/Thermal Elements/Thermal Reference  Q_Log=off  LocalVarNames=|Q  LocalVarDescs=|Q  LocalVarLogging=[]
  Ps : PMIOPort  Tag=PMCPort  Port=1  Side=Left
  H : PMIOPort  Tag=PMCPort  Port=2  Side=Left
  Kt : PMIOPort  Tag=PMCPort  Port=3  Side=Right
  T : PMIOPort  Tag=PMCPort  Port=4  Side=Right
  connections:
  Ideal Heat Flow Source/RConn1 -- Ps/RConn1
  Kt/RConn1 -- Kt as a function of temperature/RConn1
  Battery thermal mass/LConn1 -- Ideal Heat Flow Source/LConn1 -- Ideal Temperature Sensor/LConn1 -- H/RConn1
  Thermal Reference1/LConn1 -- Ideal Heat Flow Source/RConn2
  T/RConn1 -- Kt as a function of temperature/LConn1 -- Ideal Temperature Sensor/RConn2
  Ideal Temperature Sensor/RConn1 -- Thermal Reference2/LConn1

== system EVdemo_6/Battery/Cells/Battery cell6/Thermal Model ==
  Battery thermal mass : fl_lib/Thermal/Thermal Elements/Thermal Mass  mass=1 kg  sp_heat=HEV_Param.Battery_Cell.Ctheta J/kg/K  init_temp=HEV_Param.Battery_Cell.theta_init+273 K  Q_Log=off  LocalVarNames=|heat_flow|temperature  LocalVarDescs=|Heat flow (J/s)|Mass temperature (K)  LocalVarLogging=[0 0]
  Ideal Temperature Sensor : fl_lib/Thermal/Thermal Sensors/Ideal Temperature Sensor  Qs_Log=off  Ts_Log=off  LocalVarNames=|Qs|Ts  LocalVarDescs=|Qs|Ts  LocalVarLogging=[]
  Ideal Heat Flow Source : fl_lib/Thermal/Thermal Sources/Ideal Heat Flow Source  Q_Log=off  T_Log=off  LocalVarNames=|heat_flow|T_differential  LocalVarDescs=|Heat flow through the source (J/s)|Temperature differential across the source (K)  LocalVarLogging=[0 0]
  Kt as a function of temperature : fl_lib/Physical Signals/Lookup Tables/PS Lookup Table (1D)  x_t=[HEV_Param.Battery_Cell.theta_f,HEV_Param.Battery_Cell. Kt_Temps]+273  y_t=[0 HEV_Param.Battery_Cell.Kt]  interp_method=1  extrap_method=1  LocalVarLogging=[]
  Thermal Reference1 : fl_lib/Thermal/Thermal Elements/Thermal Reference  Q_Log=off  LocalVarNames=|Q  LocalVarDescs=|Q  LocalVarLogging=[]
  Thermal Reference2 : fl_lib/Thermal/Thermal Elements/Thermal Reference  Q_Log=off  LocalVarNames=|Q  LocalVarDescs=|Q  LocalVarLogging=[]
  Ps : PMIOPort  Tag=PMCPort  Port=1  Side=Left
  H : PMIOPort  Tag=PMCPort  Port=2  Side=Left
  Kt : PMIOPort  Tag=PMCPort  Port=3  Side=Right
  T : PMIOPort  Tag=PMCPort  Port=4  Side=Right
  connections:
  Ideal Heat Flow Source/RConn1 -- Ps/RConn1
  Kt/RConn1 -- Kt as a function of temperature/RConn1
  Battery thermal mass/LConn1 -- Ideal Heat Flow Source/LConn1 -- Ideal Temperature Sensor/LConn1 -- H/RConn1
  Thermal Reference1/LConn1 -- Ideal Heat Flow Source/RConn2
  T/RConn1 -- Kt as a function of temperature/LConn1 -- Ideal Temperature Sensor/RConn2
  Ideal Temperature Sensor/RConn1 -- Thermal Reference2/LConn1

== system EVdemo_6/Battery/Cells/Battery cell7/Thermal Model ==
  Battery thermal mass : fl_lib/Thermal/Thermal Elements/Thermal Mass  mass=1 kg  sp_heat=HEV_Param.Battery_Cell.Ctheta J/kg/K  init_temp=HEV_Param.Battery_Cell.theta_init+273 K  Q_Log=off  LocalVarNames=|heat_flow|temperature  LocalVarDescs=|Heat flow (J/s)|Mass temperature (K)  LocalVarLogging=[0 0]
  Ideal Temperature Sensor : fl_lib/Thermal/Thermal Sensors/Ideal Temperature Sensor  Qs_Log=off  Ts_Log=off  LocalVarNames=|Qs|Ts  LocalVarDescs=|Qs|Ts  LocalVarLogging=[]
  Ideal Heat Flow Source : fl_lib/Thermal/Thermal Sources/Ideal Heat Flow Source  Q_Log=off  T_Log=off  LocalVarNames=|heat_flow|T_differential  LocalVarDescs=|Heat flow through the source (J/s)|Temperature differential across the source (K)  LocalVarLogging=[0 0]
  Kt as a function of temperature : fl_lib/Physical Signals/Lookup Tables/PS Lookup Table (1D)  x_t=[HEV_Param.Battery_Cell.theta_f,HEV_Param.Battery_Cell. Kt_Temps]+273  y_t=[0 HEV_Param.Battery_Cell.Kt]  interp_method=1  extrap_method=1  LocalVarLogging=[]
  Thermal Reference1 : fl_lib/Thermal/Thermal Elements/Thermal Reference  Q_Log=off  LocalVarNames=|Q  LocalVarDescs=|Q  LocalVarLogging=[]
  Thermal Reference2 : fl_lib/Thermal/Thermal Elements/Thermal Reference  Q_Log=off  LocalVarNames=|Q  LocalVarDescs=|Q  LocalVarLogging=[]
  Ps : PMIOPort  Tag=PMCPort  Port=1  Side=Left
  H : PMIOPort  Tag=PMCPort  Port=2  Side=Left
  Kt : PMIOPort  Tag=PMCPort  Port=3  Side=Right
  T : PMIOPort  Tag=PMCPort  Port=4  Side=Right
  connections:
  Ideal Heat Flow Source/RConn1 -- Ps/RConn1
  Kt/RConn1 -- Kt as a function of temperature/RConn1
  Battery thermal mass/LConn1 -- Ideal Heat Flow Source/LConn1 -- Ideal Temperature Sensor/LConn1 -- H/RConn1
  Thermal Reference1/LConn1 -- Ideal Heat Flow Source/RConn2
  T/RConn1 -- Kt as a function of temperature/LConn1 -- Ideal Temperature Sensor/RConn2
  Ideal Temperature Sensor/RConn1 -- Thermal Reference2/LConn1

== system EVdemo_6/Battery/Cells/Battery cell8/Thermal Model ==
  Battery thermal mass : fl_lib/Thermal/Thermal Elements/Thermal Mass  mass=1 kg  sp_heat=HEV_Param.Battery_Cell.Ctheta J/kg/K  init_temp=HEV_Param.Battery_Cell.theta_init+273 K  Q_Log=off  LocalVarNames=|heat_flow|temperature  LocalVarDescs=|Heat flow (J/s)|Mass temperature (K)  LocalVarLogging=[0 0]
  Ideal Temperature Sensor : fl_lib/Thermal/Thermal Sensors/Ideal Temperature Sensor  Qs_Log=off  Ts_Log=off  LocalVarNames=|Qs|Ts  LocalVarDescs=|Qs|Ts  LocalVarLogging=[]
  Ideal Heat Flow Source : fl_lib/Thermal/Thermal Sources/Ideal Heat Flow Source  Q_Log=off  T_Log=off  LocalVarNames=|heat_flow|T_differential  LocalVarDescs=|Heat flow through the source (J/s)|Temperature differential across the source (K)  LocalVarLogging=[0 0]
  Kt as a function of temperature : fl_lib/Physical Signals/Lookup Tables/PS Lookup Table (1D)  x_t=[HEV_Param.Battery_Cell.theta_f,HEV_Param.Battery_Cell. Kt_Temps]+273  y_t=[0 HEV_Param.Battery_Cell.Kt]  interp_method=1  extrap_method=1  LocalVarLogging=[]
  Thermal Reference1 : fl_lib/Thermal/Thermal Elements/Thermal Reference  Q_Log=off  LocalVarNames=|Q  LocalVarDescs=|Q  LocalVarLogging=[]
  Thermal Reference2 : fl_lib/Thermal/Thermal Elements/Thermal Reference  Q_Log=off  LocalVarNames=|Q  LocalVarDescs=|Q  LocalVarLogging=[]
  Ps : PMIOPort  Tag=PMCPort  Port=1  Side=Left
  H : PMIOPort  Tag=PMCPort  Port=2  Side=Left
  Kt : PMIOPort  Tag=PMCPort  Port=3  Side=Right
  T : PMIOPort  Tag=PMCPort  Port=4  Side=Right
  connections:
  Ideal Heat Flow Source/RConn1 -- Ps/RConn1
  Kt/RConn1 -- Kt as a function of temperature/RConn1
  Battery thermal mass/LConn1 -- Ideal Heat Flow Source/LConn1 -- Ideal Temperature Sensor/LConn1 -- H/RConn1
  Thermal Reference1/LConn1 -- Ideal Heat Flow Source/RConn2
  T/RConn1 -- Kt as a function of temperature/LConn1 -- Ideal Temperature Sensor/RConn2
  Ideal Temperature Sensor/RConn1 -- Thermal Reference2/LConn1

== system EVdemo_6/Battery/Cells/Battery cell9/Thermal Model ==
  Battery thermal mass : fl_lib/Thermal/Thermal Elements/Thermal Mass  mass=1 kg  sp_heat=HEV_Param.Battery_Cell.Ctheta J/kg/K  init_temp=HEV_Param.Battery_Cell.theta_init+273 K  Q_Log=off  LocalVarNames=|heat_flow|temperature  LocalVarDescs=|Heat flow (J/s)|Mass temperature (K)  LocalVarLogging=[0 0]
  Ideal Temperature Sensor : fl_lib/Thermal/Thermal Sensors/Ideal Temperature Sensor  Qs_Log=off  Ts_Log=off  LocalVarNames=|Qs|Ts  LocalVarDescs=|Qs|Ts  LocalVarLogging=[]
  Ideal Heat Flow Source : fl_lib/Thermal/Thermal Sources/Ideal Heat Flow Source  Q_Log=off  T_Log=off  LocalVarNames=|heat_flow|T_differential  LocalVarDescs=|Heat flow through the source (J/s)|Temperature differential across the source (K)  LocalVarLogging=[0 0]
  Kt as a function of temperature : fl_lib/Physical Signals/Lookup Tables/PS Lookup Table (1D)  x_t=[HEV_Param.Battery_Cell.theta_f,HEV_Param.Battery_Cell. Kt_Temps]+273  y_t=[0 HEV_Param.Battery_Cell.Kt]  interp_method=1  extrap_method=1  LocalVarLogging=[]
  Thermal Reference1 : fl_lib/Thermal/Thermal Elements/Thermal Reference  Q_Log=off  LocalVarNames=|Q  LocalVarDescs=|Q  LocalVarLogging=[]
  Thermal Reference2 : fl_lib/Thermal/Thermal Elements/Thermal Reference  Q_Log=off  LocalVarNames=|Q  LocalVarDescs=|Q  LocalVarLogging=[]
  Ps : PMIOPort  Tag=PMCPort  Port=1  Side=Left
  H : PMIOPort  Tag=PMCPort  Port=2  Side=Left
  Kt : PMIOPort  Tag=PMCPort  Port=3  Side=Right
  T : PMIOPort  Tag=PMCPort  Port=4  Side=Right
  connections:
  Ideal Heat Flow Source/RConn1 -- Ps/RConn1
  Kt/RConn1 -- Kt as a function of temperature/RConn1
  Battery thermal mass/LConn1 -- Ideal Heat Flow Source/LConn1 -- Ideal Temperature Sensor/LConn1 -- H/RConn1
  Thermal Reference1/LConn1 -- Ideal Heat Flow Source/RConn2
  T/RConn1 -- Kt as a function of temperature/LConn1 -- Ideal Temperature Sensor/RConn2
  Ideal Temperature Sensor/RConn1 -- Thermal Reference2/LConn1

== system EVdemo_6/Battery/Cells/Measurements/Calculate battery power & charge ==
  -1/(60*60) : fl_lib/Physical Signals/Functions/PS Gain  gain=-1/(60*60)  LocalVarLogging=[]
  Initial charge Ah0 : Integrator  InitialCondition=HEV_Param.Battery_Sys.Maximum_Capacity
  PS Product : fl_lib/Physical Signals/Functions/PS Product  LocalVarLogging=[]
  PS Product1 : fl_lib/Physical Signals/Functions/PS Product  LocalVarLogging=[]
  PS-Simulink Converter : nesl_utility/PS-Simulink Converter  PhysicalDomain=network_engine_domain  SubClassName=ps_output  LeftPortType=input  RightPortType=output  PseudoPeriodic=off  Frequencies=[]  Unit=W  AffineConversion=off
  PS-Simulink Converter1 : nesl_utility/PS-Simulink Converter  PhysicalDomain=network_engine_domain  SubClassName=ps_output  LeftPortType=input  RightPortType=output  PseudoPeriodic=off  Frequencies=[]  Unit=1  AffineConversion=off
  PS-Simulink Converter2 : nesl_utility/PS-Simulink Converter  PhysicalDomain=network_engine_domain  SubClassName=ps_output  LeftPortType=input  RightPortType=output  PseudoPeriodic=off  Frequencies=[]  Unit=1  AffineConversion=off
  Rbat : Gain  Gain=HEV_Param.Battery_Sys.Internal_Resistance
  Terminator : Terminator
  Terminator1 : Terminator
  W to kW : Gain  Gain=1/1000
  V : PMIOPort  Port=1  Side=Left
  I : PMIOPort  Port=2  Side=Left
  Ah : Outport
  wires:
  Rbat/1 -> Terminator1/1  "Pr_Batt"
  PS-Simulink Converter2/1 -> Rbat/1
  Initial charge Ah0/1 -> Ah/1
  PS-Simulink Converter1/1 -> Initial charge Ah0/1  "d/dt(Ah)"
  W to kW/1 -> Terminator/1  "Pe_Batt"
  PS-Simulink Converter/1 -> W to kW/1  "Battery power"
  connections:
  PS Product1/RConn1 -- PS-Simulink Converter2/LConn1
  -1/(60*60)/RConn1 -- PS-Simulink Converter1/LConn1
  PS Product1/LConn2 -- PS Product1/LConn1 -- -1/(60*60)/LConn1 -- I/RConn1 -- PS Product/LConn2
  V/RConn1 -- PS Product/LConn1
  PS Product/RConn1 -- PS-Simulink Converter/LConn1

== system EVdemo_6/Battery/Generic/Measurements/Calculate battery power & charge ==
  -1/(60*60) : fl_lib/Physical Signals/Functions/PS Gain  gain=-1/(60*60)  LocalVarLogging=[]
  Initial charge Ah0 : Integrator  InitialCondition=HEV_Param.Battery_Sys.Maximum_Capacity
  PS Product : fl_lib/Physical Signals/Functions/PS Product  LocalVarLogging=[]
  PS Product1 : fl_lib/Physical Signals/Functions/PS Product  LocalVarLogging=[]
  PS-Simulink Converter : nesl_utility/PS-Simulink Converter  PhysicalDomain=network_engine_domain  SubClassName=ps_output  LeftPortType=input  RightPortType=output  PseudoPeriodic=off  Frequencies=[]  Unit=W  AffineConversion=off
  PS-Simulink Converter1 : nesl_utility/PS-Simulink Converter  PhysicalDomain=network_engine_domain  SubClassName=ps_output  LeftPortType=input  RightPortType=output  PseudoPeriodic=off  Frequencies=[]  Unit=1  AffineConversion=off
  PS-Simulink Converter2 : nesl_utility/PS-Simulink Converter  PhysicalDomain=network_engine_domain  SubClassName=ps_output  LeftPortType=input  RightPortType=output  PseudoPeriodic=off  Frequencies=[]  Unit=1  AffineConversion=off
  Rbat : Gain  Gain=HEV_Param.Battery_Sys.Internal_Resistance
  Terminator : Terminator
  Terminator1 : Terminator
  W to kW : Gain  Gain=1/1000
  V : PMIOPort  Port=1  Side=Left
  I : PMIOPort  Port=2  Side=Left
  Ah : Outport
  wires:
  PS-Simulink Converter/1 -> W to kW/1  "Battery power"
  W to kW/1 -> Terminator/1  "Pe_Batt"
  PS-Simulink Converter1/1 -> Initial charge Ah0/1  "d/dt(Ah)"
  Initial charge Ah0/1 -> Ah/1
  PS-Simulink Converter2/1 -> Rbat/1
  Rbat/1 -> Terminator1/1  "Pr_Batt"
  connections:
  PS Product/RConn1 -- PS-Simulink Converter/LConn1
  V/RConn1 -- PS Product/LConn1
  PS Product/LConn2 -- I/RConn1 -- -1/(60*60)/LConn1 -- PS Product1/LConn1 -- PS Product1/LConn2
  -1/(60*60)/RConn1 -- PS-Simulink Converter1/LConn1
  PS Product1/RConn1 -- PS-Simulink Converter2/LConn1

== system EVdemo_6/Battery/Generic1/Measurements/Calculate battery power & charge ==
  -1/(60*60) : fl_lib/Physical Signals/Functions/PS Gain  gain=-1/(60*60)  LocalVarLogging=[]
  Initial charge Ah0 : Integrator  InitialCondition=HEV_Param.Battery_Sys.Maximum_Capacity
  PS Product : fl_lib/Physical Signals/Functions/PS Product  LocalVarLogging=[]
  PS Product1 : fl_lib/Physical Signals/Functions/PS Product  LocalVarLogging=[]
  PS-Simulink Converter : nesl_utility/PS-Simulink Converter  PhysicalDomain=network_engine_domain  SubClassName=ps_output  LeftPortType=input  RightPortType=output  PseudoPeriodic=off  Frequencies=[]  Unit=W  AffineConversion=off
  PS-Simulink Converter1 : nesl_utility/PS-Simulink Converter  PhysicalDomain=network_engine_domain  SubClassName=ps_output  LeftPortType=input  RightPortType=output  PseudoPeriodic=off  Frequencies=[]  Unit=1  AffineConversion=off
  PS-Simulink Converter2 : nesl_utility/PS-Simulink Converter  PhysicalDomain=network_engine_domain  SubClassName=ps_output  LeftPortType=input  RightPortType=output  PseudoPeriodic=off  Frequencies=[]  Unit=1  AffineConversion=off
  Rbat : Gain  Gain=HEV_Param.Battery_Sys.Internal_Resistance
  Terminator : Terminator
  Terminator1 : Terminator
  W to kW : Gain  Gain=1/1000
  V : PMIOPort  Port=1  Side=Left
  I : PMIOPort  Port=2  Side=Left
  Ah : Outport
  wires:
  Rbat/1 -> Terminator1/1  "Pr_Batt"
  PS-Simulink Converter2/1 -> Rbat/1
  Initial charge Ah0/1 -> Ah/1
  PS-Simulink Converter1/1 -> Initial charge Ah0/1  "d/dt(Ah)"
  W to kW/1 -> Terminator/1  "Pe_Batt"
  PS-Simulink Converter/1 -> W to kW/1  "Battery power"
  connections:
  PS Product1/RConn1 -- PS-Simulink Converter2/LConn1
  -1/(60*60)/RConn1 -- PS-Simulink Converter1/LConn1
  PS Product1/LConn2 -- PS Product1/LConn1 -- -1/(60*60)/LConn1 -- I/RConn1 -- PS Product/LConn2
  V/RConn1 -- PS Product/LConn1
  PS Product/RConn1 -- PS-Simulink Converter/LConn1

== system EVdemo_6/Battery/Predefined/GF1/SOC Offset ==
  note: For control logic to work consistently
      | for all versions, SOC% must be scaled
  In1 : Inport
  Bus Creator : BusCreator
  Bus Selector : BusSelector  OutputSignals=SOC (%)
  Bus Selector1 : BusSelector  OutputSignals=Current (A),Voltage (V)
  Gain : Gain  Gain=100/HEV_Param.Battery_Det.Initial_SOC
  Gain1 : Gain  Gain=-1/(60*60)
  Initial charge Ah0 : Integrator  InitialCondition=HEV_Param.Battery_Det.Rated_Capacity*HEV_Param.Battery_Det.Initial_SOC/100
  Out1 : Outport
  wires:
  Initial charge Ah0/1 -> Bus Creator/1  "Batt_Ah"
  Gain1/1 -> Initial charge Ah0/1
  Bus Creator/1 -> Out1/1
  Bus Selector1/2 -> Bus Creator/3  "<Voltage (V)>"
  Gain/1 -> Bus Creator/4  "SOC (%)"
  Bus Selector1/1 -> Gain1/1, Bus Creator/2  "<Current (A)>"
  Bus Selector/1 -> Gain/1  "<SOC (%)>"
  In1/1 -> Bus Selector1/1, Bus Selector/1
